simulink model "Model"  (R2021b)
settings: Solver=VariableStepAuto  StartTime=0.0  StopTime=1650  RelTol=1e-3
settings Model: Creator=aman  LastModifiedBy=aman

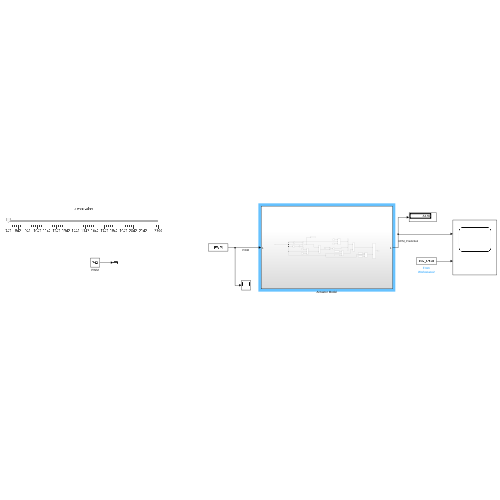
[thumbnail: Simulink's stored preview of the top-level diagram]
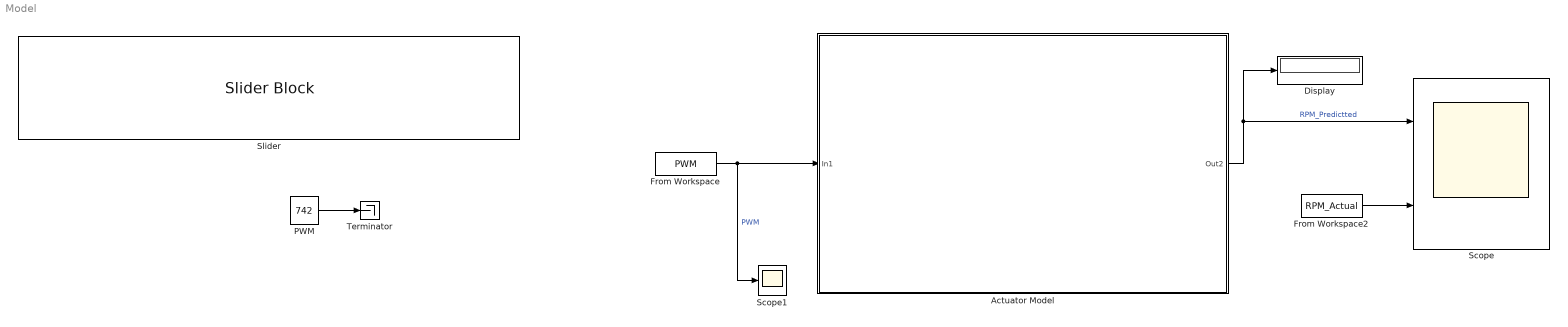
== system Model ==
  Actuator Model : Subsystem
  Display : Display
  From Workspace : FromWorkspace  VariableName=PWM
  From Workspace2 : FromWorkspace  VariableName=RPM_Actual
  PWM : Constant  Value=742
  Scope : Scope  NumInputPorts=2
  Scope1 : Scope
  Slider : SliderBlock  ScaleMin=742  ScaleMax=2300
  Terminator : Terminator
  wires:
  Actuator Model/1(Out2) -> Display/1, Scope/1  "RPM_Predictted"
  PWM/1 -> Terminator/1
  From Workspace/1 -> Scope1/1, Actuator Model/1(In1)  "PWM"
  From Workspace2/1 -> Scope/2

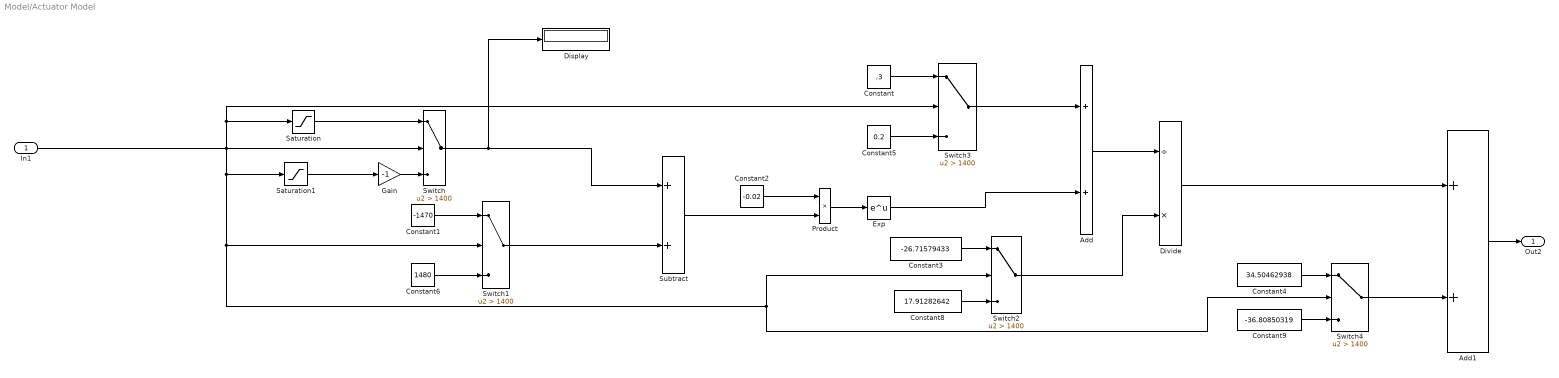
== system Model/Actuator Model ==
  In1 : Inport
  Add : Sum
  Add1 : Sum
  Constant : Constant  Value=.3
  Constant1 : Constant  Value=-1470
  Constant2 : Constant  Value=-0.02
  Constant3 : Constant  Value=-26.71579433
  Constant4 : Constant  Value=34.50462938
  Constant5 : Constant  Value=0.2
  Constant6 : Constant  Value=1480
  Constant8 : Constant  Value=17.91282642
  Constant9 : Constant  Value=-36.80850319
  Display : Display
  Divide : Product  Inputs=/*
  Exp : Math  SaturateOnIntegerOverflow=on
  Gain : Gain  Gain=-1
  Product : Product
  Saturation : Saturate  UpperLimit=2300  LowerLimit=1508
  Saturation1 : Saturate  UpperLimit=1400  LowerLimit=742
  Subtract : Sum
  Switch{,1..4} (5 alike) : Switch  Criteria=u2 > Threshold  Threshold=1400
  Out2 : Outport
  wires:
  Divide/1 -> Add1/1
  Add/1 -> Divide/1
  Exp/1 -> Add/2
  Product/1 -> Exp/1
  Constant2/1 -> Product/1
  Subtract/1 -> Product/2
  In1/1 -> Switch/2, Switch3/2, Saturation/1, Switch4/2, Switch2/2, Switch1/2, Saturation1/1
  Gain/1 -> Switch/3
  Switch/1 -> Display/1, Subtract/1
  Constant1/1 -> Switch1/1
  Constant6/1 -> Switch1/3
  Saturation/1 -> Switch/1
  Saturation1/1 -> Gain/1
  Switch1/1 -> Subtract/2
  Constant3/1 -> Switch2/1
  Constant8/1 -> Switch2/3
  Switch2/1 -> Divide/2
  Constant/1 -> Switch3/1
  Constant5/1 -> Switch3/3
  Switch3/1 -> Add/1
  Constant4/1 -> Switch4/1
  Constant9/1 -> Switch4/3
  Switch4/1 -> Add1/2
  Add1/1 -> Out2/1
